simulink model "tank_mod_"  (R2020b)
settings: Solver=VariableStepAuto  StartTime=0.0  StopTime=10.0  RelTol=1e-3
values from neighbouring files (symbols this model uses):
  A = [A11 A12 A13 ; A21 A22 A23 ; A31 A32 A33 ]    [tank_mod.m]
  B = [B11 B12 ; B21 B22 ;B31 B32 ]    [tank_mod.m]
  C = [7 7 7]    [deadline_ej.m]    (also in deadline_min.m = 10*[0.3 3 3]; deadline_motonic.m = [0.6 0.375 0.6]'; deadline_tesis.m = [1.5 5 0.3]; tank_mod.m = eye(3))
  K1 = [21.6 3 -5; 2.9 19 -4]*10e-4    [tank_mod.m]
  K2 = [-0.95 -0.32; -0.3 -0.91]*10e-4    [tank_mod.m]
  tm = 0.001    [tank_mod.m]
  tm2 = 0.005    [tank_mod.m]
libraries: pid_lib x1
settings Model: Creator=Acer  LastModifiedBy=Acer

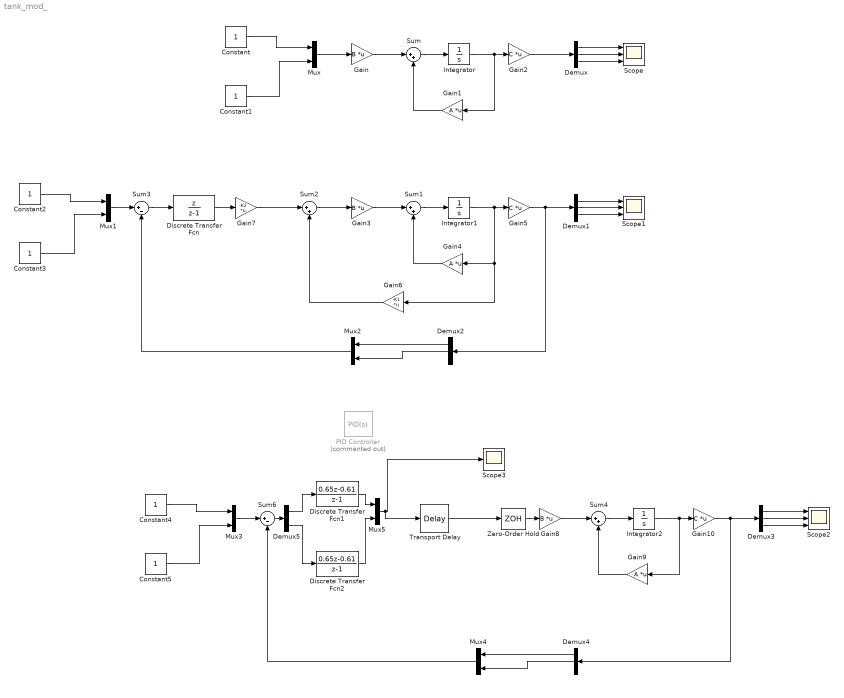
== system tank_mod_ ==
  Constant{,1..5} (6 alike) : Constant
  Demux{,1..4} (5 alike) : Demux  Outputs=3
  Demux5 : Demux  Outputs=2
  Discrete Transfer Fcn : DiscreteTransferFcn  Numerator=[1 0]  Denominator=[1 -1]  SampleTime=tm
  Discrete Transfer Fcn1 : DiscreteTransferFcn  Numerator=[0.65 -0.61]  Denominator=[1 -1]  SampleTime=tm2
  Discrete Transfer Fcn2 : DiscreteTransferFcn  Numerator=[0.65 -0.61]  Denominator=[1 -1]  SampleTime=tm2
  Gain : Gain  Gain=B  Multiplication=Matrix(K*u)
  Gain1 : Gain  Gain=A  Multiplication=Matrix(K*u)
  Gain10 : Gain  Gain=C  Multiplication=Matrix(K*u)
  Gain2 : Gain  Gain=C  Multiplication=Matrix(K*u)
  Gain3 : Gain  Gain=B  Multiplication=Matrix(K*u)
  Gain4 : Gain  Gain=A  Multiplication=Matrix(K*u)
  Gain5 : Gain  Gain=C  Multiplication=Matrix(K*u)
  Gain6 : Gain  Gain=-K1  Multiplication=Matrix(K*u)
  Gain7 : Gain  Gain=-K2  Multiplication=Matrix(K*u)
  Gain8 : Gain  Gain=B  Multiplication=Matrix(K*u)
  Gain9 : Gain  Gain=A  Multiplication=Matrix(K*u)
  Integrator : Integrator
  Integrator1 : Integrator
  Integrator2 : Integrator
  Mux{,1..5} (6 alike) : Mux  Inputs=2
  PID Controller : pid_lib/PID Controller  Commented=on  Controller=PID  Form=Parallel  TimeDomain=Continuous-time  UseExternalTs=off  SampleTime=0.01  IntegratorMethod=Forward Euler  FilterMethod=Forward Euler  ControllerParametersSource=internal  P=0.65  I=8  D=0  UseFilter=on  N=58.4444959725298  TunerSelectOption=Transfer Function Based (PID Tuner App)  InitialConditionSource=internal  InitialConditionForIntegrator=0  InitialConditionForFilter=0  DifferentiatorICPrevScaledInput=0  ExternalReset=none  TrackingMode=off  Kt=1  LimitOutput=off  SatLimitsSource=internal  UpperSaturationLimit=inf  LowerSaturationLimit=-inf  LinearizeAsGain=on  AntiWindupMode=none  Kb=1  POutMin=[]  POutMax=[]  IOutMin=[]  IOutMax=[]  DOutMin=[]  DOutMax=[]  NOutMin=[]  NOutMax=[]  SumOutMin=[]  SumOutMax=[]  SaturationOutMin=[]  SaturationOutMax=[]  PParamMin=[]  PParamMax=[]  IParamMin=[]  IParamMax=[]  DParamMin=[]  DParamMax=[]  NParamMin=[]  NParamMax=[]  KbParamMin=[]  KbParamMax=[]  KtParamMin=[]  KtParamMax=[]  KbOutMin=[]  KbOutMax=[]  KtOutMin=[]  KtOutMax=[]  IntegratorOutMin=[]  IntegratorOutMax=[]  FilterOutMin=[]  FilterOutMax=[]  SumI1OutMin=[]  SumI1OutMax=[]  SumI2OutMin=[]  SumI2OutMax=[]  SumI3OutMin=[]  SumI3OutMax=[]  SumI4OutMin=[]  SumI4OutMax=[]  SumDOutMin=[]  SumDOutMax=[]  DifferentiatorOutMin=[]  DifferentiatorOutMax=[]  FilterDiffOutCoefMin=[]  FilterDiffOutCoefMax=[]  ReciprocalOutMin=[]  ReciprocalOutMax=[]  SumDenOutMin=[]  SumDenOutMax=[]  SumNumOutMin=[]  SumNumOutMax=[]  DivideOutMin=[]  DivideOutMax=[]  UdiffTsProdOutMin=[]  UdiffTsProdOutMax=[]  NTsProdOutMin=[]  NTsProdOutMax=[]  UintegralTsProdOutMin=[]  UintegralTsProdOutMax=[]  UngainTsProdOutMin=[]  UngainTsProdOutMax=[]  IntegratorContinuousStateAttributes=''  IntegratorStateMustResolveToSignalObject=off  IntegratorRTWStateStorageClass=Auto  FilterContinuousStateAttributes=''  FilterStateMustResolveToSignalObject=off  FilterRTWStateStorageClass=Auto  ParallelPVariant=InternalParameters  IdealPVariant=Disabled  IVariant=InternalParameters  DVariant=InternalParameters  IntegratorVariant=Continuous  SatVariant=Disabled  AWVariant=Passthrough  PCopyVariant=Disabled  TRVariant=Disabled  FdbkBlocksVariant=Forward  IdealPFdbkVariant=Disabled  SatFdbkVariant=Disabled  DerivativeFilterVariant=ContFilter  NVariant=InternalParameters  NCopyVariant=Disabled  FilterICVariant=InternalICsFilter  IntegratorICVariant=InternalICs  ExternalResetVariant=Disabled  TRSumVariant=Passthrough  SumFdbkVariant=Disabled  SumVariant=Sum_PID  TsampFilterVariant=InternalTs  TsampNgainVariant=Passthrough  TsampIntegralVariant=Passthrough  ExternalSaturationOutDataTypeStr=Inherit: Same as second input
  Scope : Scope  NumInputPorts=3
  Scope1 : Scope  NumInputPorts=3
  Scope2 : Scope  NumInputPorts=3
  Scope3 : Scope
  Sum{,1..2,4} (4 alike) : Sum  Inputs=|++
  Sum3 : Sum  Inputs=|+-
  Sum6 : Sum  Inputs=|+-
  Transport Delay : TransportDelay  DelayTime=tm2*5
  Zero-Order Hold : ZeroOrderHold  SampleTime=tm
  wires:
  Constant/1 -> Mux/1
  Constant1/1 -> Mux/2
  Mux/1 -> Gain/1
  Gain2/1 -> Demux/1
  Gain/1 -> Sum/1
  Sum/1 -> Integrator/1
  Gain1/1 -> Sum/2
  Integrator/1 -> Gain2/1, Gain1/1
  Demux/1 -> Scope/1
  Demux/2 -> Scope/2
  Demux/3 -> Scope/3
  Demux1/1 -> Scope1/1
  Gain5/1 -> Demux2/1, Demux1/1
  Gain4/1 -> Sum1/2
  Sum1/1 -> Integrator1/1
  Gain3/1 -> Sum1/1
  Integrator1/1 -> Gain5/1, Gain6/1, Gain4/1
  Demux1/3 -> Scope1/3
  Demux1/2 -> Scope1/2
  Sum2/1 -> Gain3/1
  Gain6/1 -> Sum2/2
  Gain7/1 -> Sum2/1
  Constant2/1 -> Mux1/1
  Constant3/1 -> Mux1/2
  Mux1/1 -> Sum3/1
  Demux2/1 -> Mux2/1
  Demux2/2 -> Mux2/2
  Mux2/1 -> Sum3/2
  Sum3/1 -> Discrete Transfer Fcn/1
  Discrete Transfer Fcn/1 -> Gain7/1
  Constant5/1 -> Mux3/2
  Mux3/1 -> Sum6/1
  Demux4/2 -> Mux4/2
  Sum4/1 -> Integrator2/1
  Demux4/1 -> Mux4/1
  Mux4/1 -> Sum6/2
  Gain8/1 -> Sum4/1
  Gain10/1 -> Demux4/1, Demux3/1
  Integrator2/1 -> Gain10/1, Gain9/1
  Gain9/1 -> Sum4/2
  Constant4/1 -> Mux3/1
  Demux3/3 -> Scope2/3
  Demux3/1 -> Scope2/1
  Demux3/2 -> Scope2/2
  Sum6/1 -> Demux5/1
  Demux5/1 -> Discrete Transfer Fcn1/1
  Demux5/2 -> Discrete Transfer Fcn2/1
  Discrete Transfer Fcn1/1 -> Mux5/1
  Discrete Transfer Fcn2/1 -> Mux5/2
  Mux5/1 -> Transport Delay/1, Scope3/1
  Zero-Order Hold/1 -> Gain8/1
  Transport Delay/1 -> Zero-Order Hold/1
